simulink model "cylinderMechanical"  (R2019b)
settings: Solver=VariableStepAuto  StartTime=0.0  StopTime=5  RelTol=1e-3
undefined symbols (not defined in the file): B_hs, B_ks, beta, Cp, Cv, F_L, Fc, gamma, K_hs, K_ks, L, M, M_L, P_0, p_A0, p_B0, R, S_0, S_A, S_B, T, V_0A, V_0B, x0
libraries: simulink x2
settings Model: Creator=artof  LastModifiedBy=artof

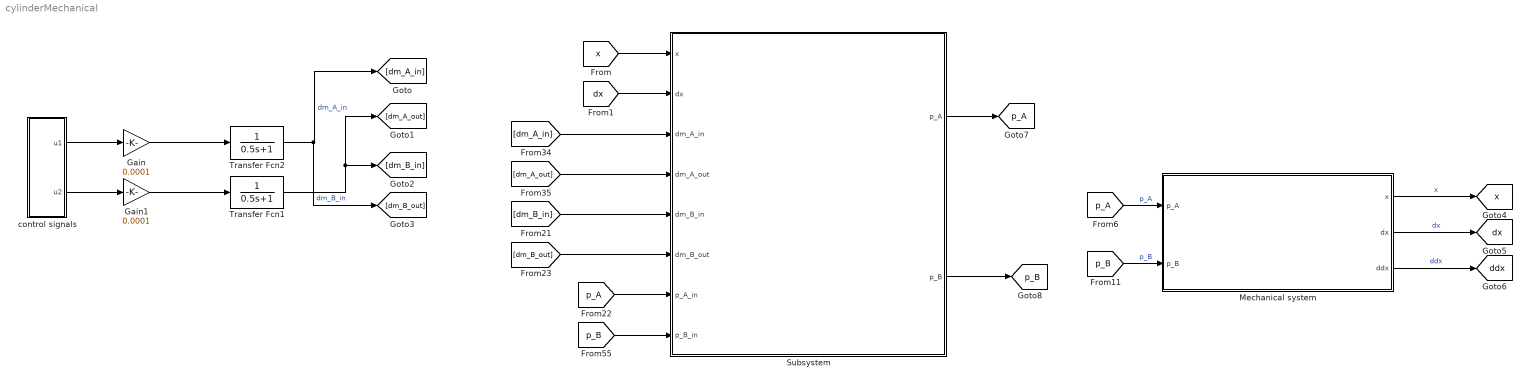
== system cylinderMechanical ==
  Gain : Gain  Gain=0.0001
  Gain1 : Gain  Gain=0.0001
  Mechanical system : Subsystem
  Subsystem : Subsystem
  Transfer Fcn1 : TransferFcn  Denominator=[0.5 1]
  Transfer Fcn2 : TransferFcn  Denominator=[0.5 1]
  control signals : Subsystem
  tag scope: ddx=global, dx=global, p_A=global, p_B=global, x=global
  wires:
  Mechanical system/2(dx) -> [dx]  "dx"
  [p_A] -> Mechanical system/1(p_A)  "p_A"
  [p_B] -> Mechanical system/2(p_B)  "p_B"
  Mechanical system/3(ddx) -> [ddx]  "ddx"
  Mechanical system/1(x) -> [x]  "x"
  Subsystem/1(p_A) -> [p_A]
  Subsystem/2(p_B) -> [p_B]
  [x] -> Subsystem/1(x)
  [dx] -> Subsystem/2(dx)
  [dm_A_out] -> Subsystem/4(dm_A_out)
  [dm_A_in] -> Subsystem/3(dm_A_in)
  [dm_B_in] -> Subsystem/5(dm_B_in)
  [dm_B_out] -> Subsystem/6(dm_B_out)
  [p_B] -> Subsystem/8(p_B_in)
  [p_A] -> Subsystem/7(p_A_in)
  control signals/2(u2) -> Gain1/1
  control signals/1(u1) -> Gain/1
  Transfer Fcn2/1 -> [dm_B_out], [dm_A_in]  "dm_A_in"
  Transfer Fcn1/1 -> [dm_A_out], [dm_B_in]  "dm_B_in"
  Gain/1 -> Transfer Fcn2/1
  Gain1/1 -> Transfer Fcn1/1

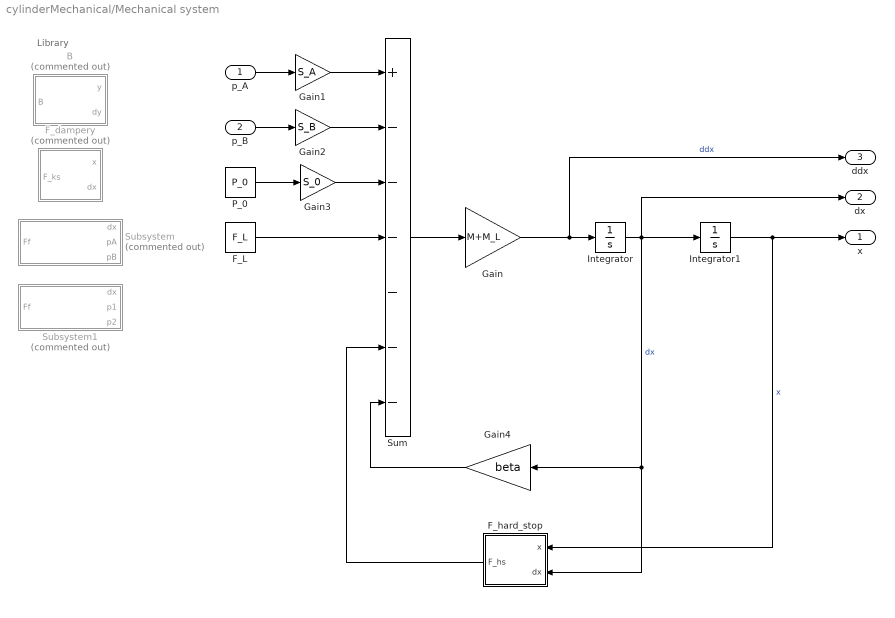
== system cylinderMechanical/Mechanical system ==
  note: Library
  p_A : Inport
  p_B : Inport  Port=2
  B : MATLAB Function  Commented=on  TreatAsAtomicUnit=on
  F_L : Constant  Value=F_L
  F_dampery : Subsystem  Commented=on
  F_hard_stop : Subsystem
  Gain : Gain  Gain=M+M_L
  Gain1 : Gain  Gain=S_A
  Gain2 : Gain  Gain=S_B
  Gain3 : Gain  Gain=S_0
  Gain4 : Gain  Gain=beta
  Integrator : Integrator
  Integrator1 : Integrator  InitialCondition=x0
  P_0 : Constant  Value=P_0
  Subsystem : Subsystem  Commented=on
  Subsystem1 : Subsystem  Commented=on
  Sum : Sum  Inputs=+------
  x : Outport
  dx : Outport  Port=2
  ddx : Outport  Port=3
  wires:
  p_A/1 -> Gain1/1
  Gain/1 -> ddx/1, Integrator/1  "ddx"
  Sum/1 -> Gain/1
  F_L/1 -> Sum/4
  P_0/1 -> Gain3/1
  Gain3/1 -> Sum/3
  Integrator/1 -> dx/1, F_hard_stop/2(dx), Gain4/1, Integrator1/1  "dx"
  Integrator1/1 -> x/1, F_hard_stop/1(x)  "x"
  p_B/1 -> Gain2/1
  Gain2/1 -> Sum/2
  F_hard_stop/1(F_hs) -> Sum/6
  Gain1/1 -> Sum/1
  Gain4/1 -> Sum/7

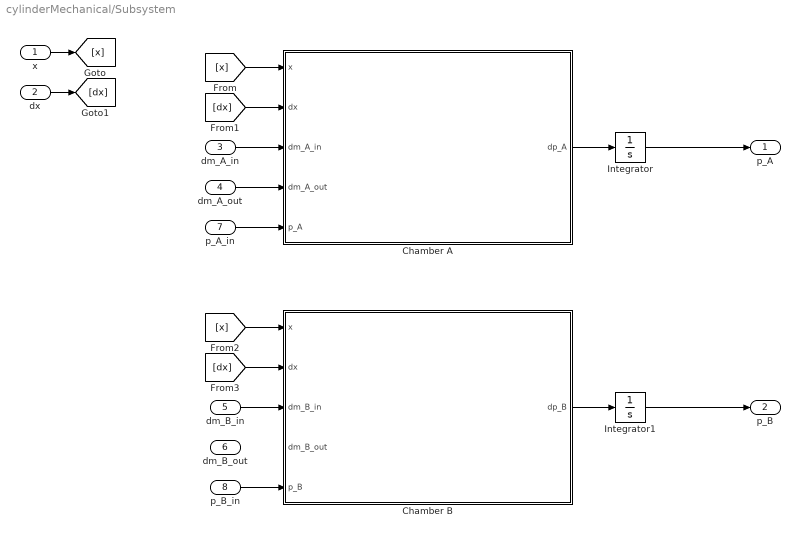
== system cylinderMechanical/Subsystem ==
  x : Inport
  dx : Inport  Port=2
  dm_A_in : Inport  Port=3
  dm_A_out : Inport  Port=4
  dm_B_in : Inport  Port=5
  dm_B_out : Inport  Port=6
  p_A_in : Inport  Port=7
  p_B_in : Inport  Port=8
  Chamber A : Subsystem
  Chamber B : Subsystem
  Integrator : Integrator  InitialCondition=p_A0
  Integrator1 : Integrator  InitialCondition=p_B0
  p_A : Outport
  p_B : Outport  Port=2
  wires:
  Chamber B/1(dp_B) -> Integrator1/1
  [x] -> Chamber A/1(x)
  Chamber A/1(dp_A) -> Integrator/1
  [dx] -> Chamber B/2(dx)
  Integrator/1 -> p_A/1
  [x] -> Chamber B/1(x)
  Integrator1/1 -> p_B/1
  [dx] -> Chamber A/2(dx)
  dx/1 -> [dx]
  x/1 -> [x]
  dm_A_in/1 -> Chamber A/3(dm_A_in)
  dm_A_out/1 -> Chamber A/4(dm_A_out)
  dm_B_in/1 -> Chamber B/3(dm_B_in)
  p_A_in/1 -> Chamber A/5(p_A)
  p_B_in/1 -> Chamber B/5(p_B)

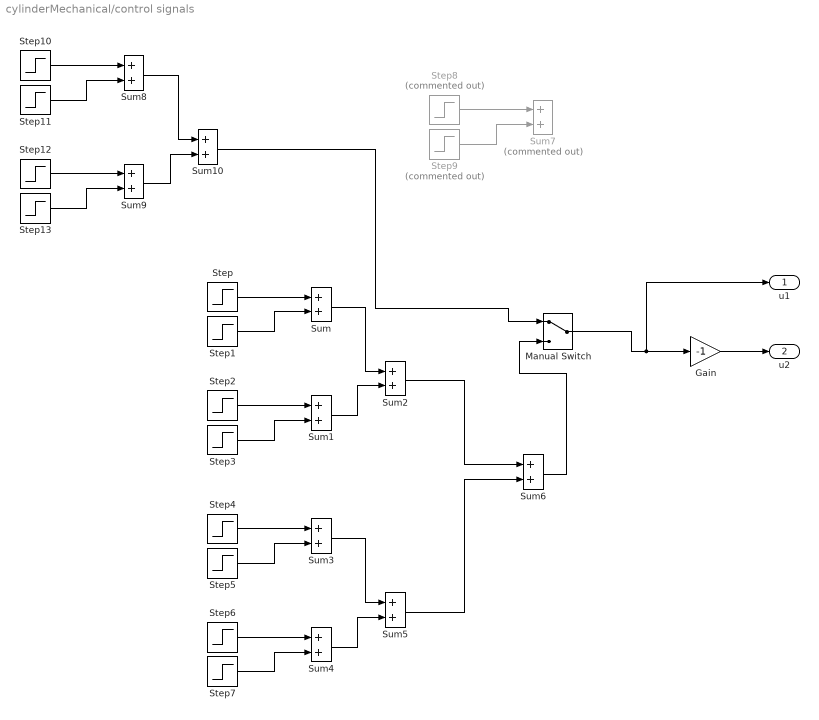
== system cylinderMechanical/control signals ==
  Gain : Gain  Gain=-1
  Manual Switch : ManualSwitch
  Step : Step  SampleTime=0
  Step1 : Step  Time=1.3  After=-1  SampleTime=0
  Step10 : Step  SampleTime=0
  Step11 : Step  Time=6  After=-1  SampleTime=0
  Step12 : Step  Time=6  After=-1  SampleTime=0
  Step13 : Step  Time=10  SampleTime=0
  Step2 : Step  Time=2  After=-1  SampleTime=0
  Step3 : Step  Time=2.3  SampleTime=0
  Step4 : Step  Time=3  SampleTime=0
  Step5 : Step  Time=3.3  After=-1  SampleTime=0
  Step6 : Step  Time=4  After=-1  SampleTime=0
  Step7 : Step  Time=4.3  SampleTime=0
  Step8 : Step  Commented=on  SampleTime=0
  Step9 : Step  Commented=on  Time=6  After=-1  SampleTime=0
  Sum{,1..6,8..10} (10 alike) : Sum
  Sum7 : Sum  Commented=on
  u1 : Outport
  u2 : Outport  Port=2
  wires:
  Gain/1 -> u2/1
  Sum/1 -> Sum2/1
  Step1/1 -> Sum/2
  Step/1 -> Sum/1
  Step3/1 -> Sum1/2
  Step2/1 -> Sum1/1
  Sum1/1 -> Sum2/2
  Sum4/1 -> Sum5/2
  Step6/1 -> Sum4/1
  Step7/1 -> Sum4/2
  Step4/1 -> Sum3/1
  Step5/1 -> Sum3/2
  Sum3/1 -> Sum5/1
  Sum5/1 -> Sum6/2
  Sum2/1 -> Sum6/1
  Sum6/1 -> Manual Switch/2
  Manual Switch/1 -> u1/1, Gain/1
  Step8/1 -> Sum7/1
  Step9/1 -> Sum7/2
  Sum10/1 -> Manual Switch/1
  Sum9/1 -> Sum10/2
  Step12/1 -> Sum9/1
  Step13/1 -> Sum9/2
  Step10/1 -> Sum8/1
  Step11/1 -> Sum8/2
  Sum8/1 -> Sum10/1

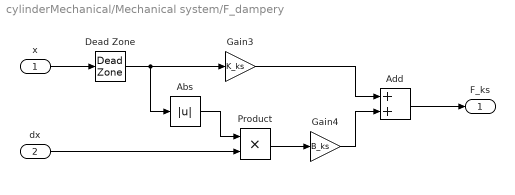
== system cylinderMechanical/Mechanical system/F_dampery ==
  x : Inport
  dx : Inport  Port=2
  Abs : Abs
  Add : Sum
  Dead Zone : DeadZone  LowerValue=0.02  UpperValue=0.180  SaturateOnIntegerOverflow=on
  Gain3 : Gain  Gain=K_ks
  Gain4 : Gain  Gain=B_ks
  Product : Product
  F_ks : Outport
  wires:
  Gain4/1 -> Add/2
  dx/1 -> Product/2
  Add/1 -> F_ks/1
  x/1 -> Dead Zone/1
  Gain3/1 -> Add/1
  Abs/1 -> Product/1
  Dead Zone/1 -> Abs/1, Gain3/1
  Product/1 -> Gain4/1

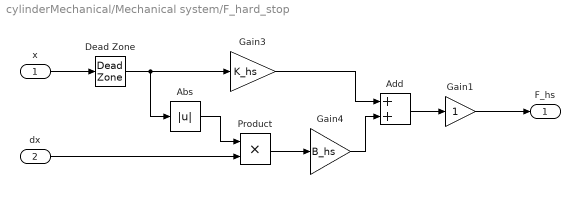
== system cylinderMechanical/Mechanical system/F_hard_stop ==
  x : Inport
  dx : Inport  Port=2
  Abs : Abs
  Add : Sum
  Dead Zone : DeadZone  LowerValue=0  UpperValue=L  SaturateOnIntegerOverflow=on
  Gain1 : Gain
  Gain3 : Gain  Gain=K_hs
  Gain4 : Gain  Gain=B_hs
  Product : Product
  F_hs : Outport
  wires:
  Product/1 -> Gain4/1
  Dead Zone/1 -> Gain3/1, Abs/1
  Abs/1 -> Product/1
  Gain3/1 -> Add/1
  x/1 -> Dead Zone/1
  Add/1 -> Gain1/1
  dx/1 -> Product/2
  Gain4/1 -> Add/2
  Gain1/1 -> F_hs/1

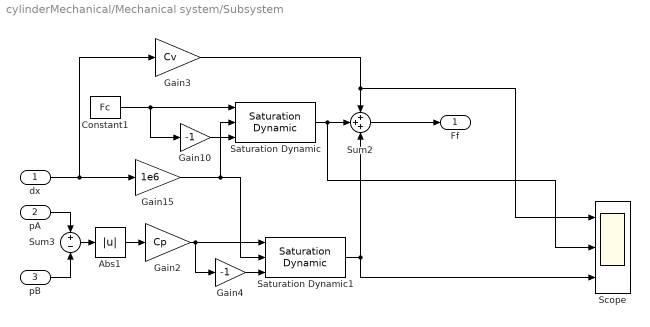
== system cylinderMechanical/Mechanical system/Subsystem ==
  dx : Inport
  pA : Inport  Port=2
  pB : Inport  Port=3
  Abs1 : Abs
  Constant1 : Constant  Value=Fc
  Gain10 : Gain  Gain=-1
  Gain15 : Gain  Gain=1e6
  Gain2 : Gain  Gain=Cp
  Gain3 : Gain  Gain=Cv
  Gain4 : Gain  Gain=-1
  Saturation Dynamic : simulink/Discontinuities/Saturation Dynamic  OutMin=[]  OutMax=[]  OutDataTypeStr=Inherit: Same as second input  OutDataType=sfix(16)  OutScaling=2^-10  DoSatur=off
  Saturation Dynamic1 : simulink/Discontinuities/Saturation Dynamic  OutMin=[]  OutMax=[]  OutDataTypeStr=Inherit: Same as second input  OutDataType=sfix(16)  OutScaling=2^-10  DoSatur=off
  Scope : Scope  NumInputPorts=3
  Sum2 : Sum  Inputs=+++
  Sum3 : Sum  Inputs=+|-
  Ff : Outport
  wires:
  Gain3/1 -> Scope/1, Sum2/1
  Gain2/1 -> Saturation Dynamic1/1, Gain4/1
  pA/1 -> Sum3/1
  dx/1 -> Gain3/1, Gain15/1
  pB/1 -> Sum3/2
  Saturation Dynamic1/1 -> Sum2/3, Scope/3
  Abs1/1 -> Gain2/1
  Sum2/1 -> Ff/1
  Gain15/1 -> Saturation Dynamic/2, Saturation Dynamic1/2
  Constant1/1 -> Saturation Dynamic/1, Gain10/1
  Gain4/1 -> Saturation Dynamic1/3
  Sum3/1 -> Abs1/1
  Gain10/1 -> Saturation Dynamic/3
  Saturation Dynamic/1 -> Scope/2, Sum2/2

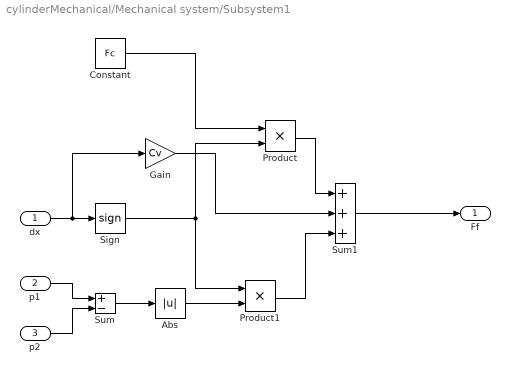
== system cylinderMechanical/Mechanical system/Subsystem1 ==
  dx : Inport
  p1 : Inport  Port=2
  p2 : Inport  Port=3
  Abs : Abs
  Constant : Constant  Value=Fc
  Gain : Gain  Gain=Cv
  Product : Product
  Product1 : Product
  Sign : Signum
  Sum : Sum  Inputs=+-
  Sum1 : Sum  Inputs=+++
  Ff : Outport
  wires:
  dx/1 -> Gain/1, Sign/1
  p2/1 -> Sum/2
  p1/1 -> Sum/1
  Sum/1 -> Abs/1
  Sign/1 -> Product/2, Product1/1
  Sum1/1 -> Ff/1
  Gain/1 -> Sum1/2
  Constant/1 -> Product/1
  Abs/1 -> Product1/2
  Product1/1 -> Sum1/3
  Product/1 -> Sum1/1

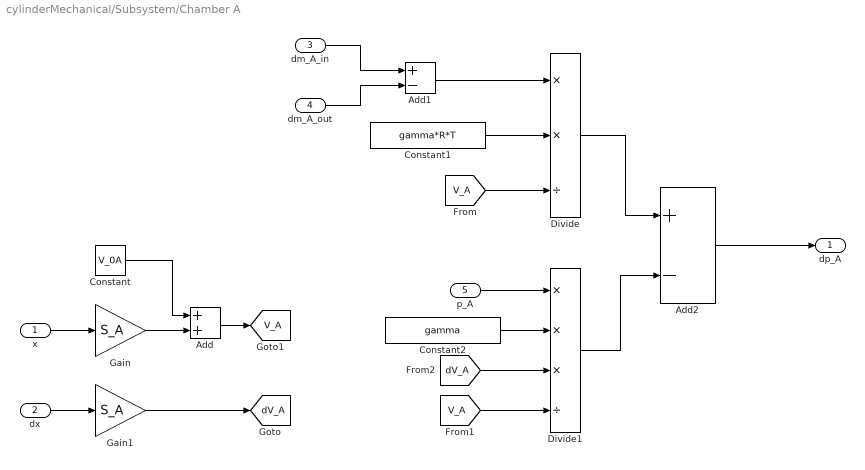
== system cylinderMechanical/Subsystem/Chamber A ==
  x : Inport
  dx : Inport  Port=2
  dm_A_in : Inport  Port=3
  dm_A_out : Inport  Port=4
  p_A : Inport  Port=5
  Add : Sum
  Add1 : Sum  Inputs=+-
  Add2 : Sum  Inputs=+-
  Constant : Constant  Value=V_0A
  Constant1 : Constant  Value=gamma*R*T
  Constant2 : Constant  Value=gamma
  Divide : Product  Inputs=**/
  Divide1 : Product  Inputs=***/
  Gain : Gain  Gain=S_A
  Gain1 : Gain  Gain=S_A
  dp_A : Outport
  tag scope: V_A=global, dV_A=global
  wires:
  x/1 -> Gain/1
  Gain/1 -> Add/2
  Constant/1 -> Add/1
  dx/1 -> Gain1/1
  Gain1/1 -> [dV_A]
  Add/1 -> [V_A]
  dm_A_out/1 -> Add1/2
  dm_A_in/1 -> Add1/1
  Add1/1 -> Divide/1
  Constant1/1 -> Divide/2
  [V_A] -> Divide/3
  Divide/1 -> Add2/1
  p_A/1 -> Divide1/1
  Constant2/1 -> Divide1/2
  [V_A] -> Divide1/4
  [dV_A] -> Divide1/3
  Divide1/1 -> Add2/2
  Add2/1 -> dp_A/1

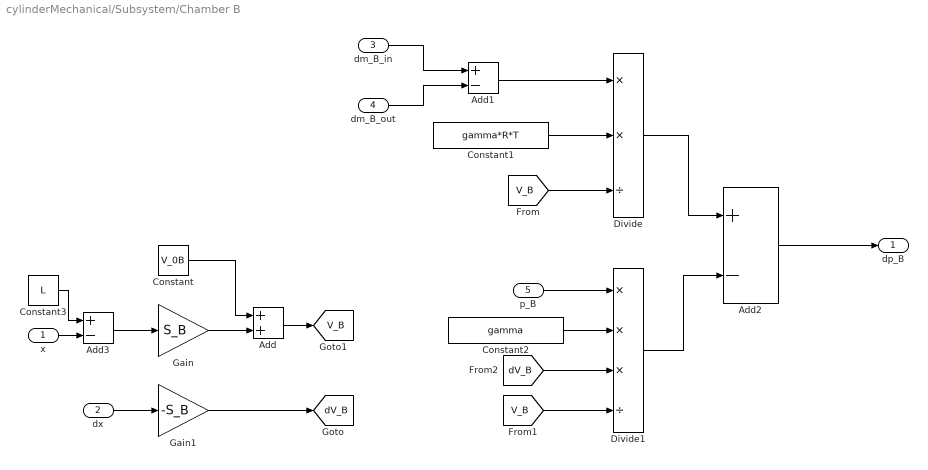
== system cylinderMechanical/Subsystem/Chamber B ==
  x : Inport
  dx : Inport  Port=2
  dm_B_in : Inport  Port=3
  dm_B_out : Inport  Port=4
  p_B : Inport  Port=5
  Add : Sum
  Add1 : Sum  Inputs=+-
  Add2 : Sum  Inputs=+-
  Add3 : Sum  Inputs=+-
  Constant : Constant  Value=V_0B
  Constant1 : Constant  Value=gamma*R*T
  Constant2 : Constant  Value=gamma
  Constant3 : Constant  Value=L
  Divide : Product  Inputs=**/
  Divide1 : Product  Inputs=***/
  Gain : Gain  Gain=S_B
  Gain1 : Gain  Gain=-S_B
  dp_B : Outport
  tag scope: V_B=global, dV_B=global
  wires:
  Add2/1 -> dp_B/1
  Divide1/1 -> Add2/2
  [dV_B] -> Divide1/3
  [V_B] -> Divide1/4
  Constant2/1 -> Divide1/2
  p_B/1 -> Divide1/1
  Divide/1 -> Add2/1
  [V_B] -> Divide/3
  Constant1/1 -> Divide/2
  Add1/1 -> Divide/1
  dm_B_in/1 -> Add1/1
  dm_B_out/1 -> Add1/2
  Add/1 -> [V_B]
  Gain1/1 -> [dV_B]
  dx/1 -> Gain1/1
  Constant/1 -> Add/1
  Gain/1 -> Add/2
  x/1 -> Add3/2
  Add3/1 -> Gain/1
  Constant3/1 -> Add3/1

== matlab function cylinderMechanical/Mechanical system/B ==
  data: y input; B output; dy input
function B = fcn(y,dy)
%global b1 b2 b_max b_min
b_max   = 0.18;    %[m]
b_min   = 0.02;    %[m]
b1      = 100;    %[kg/s]
b2      = 100;    %[kg/s]   
if y > b_max && sign(dy) > 0
    B = b1;
elseif y < b_min && sign(dy) < 0 
    B = b2;
else
    B = 0;
end
end
